simulink model "pingtai_with_control_gaijin1PIDNN3_2"  (R2014a)
settings: Solver=ode23t  StartTime=0.0  StopTime=100.0  MaxStep=1e-2  RelTol=1e-3
values from neighbouring files (symbols this model uses):
  m = 0    [cs_search.m]    (also in pso_search.m = n)
  s = new_nest(j,:)    [empty_nests.m]    (also in get_cuckoos.m = s+stepsize.*randn(size(s)); pso_search.m = newnest(i,:); simplebounds.m = ns_tmp)
undefined symbols (not defined in the file or in its folder): mpidnn, sigbuilder_block, WW, X, Y, Z
libraries: fl_lib x68, sm_lib x65, nesl_utility x65, simulink x18, sm_radial_engine_lib x8, sdl_lib x8, elec_lib x4
(part 4 of 5)

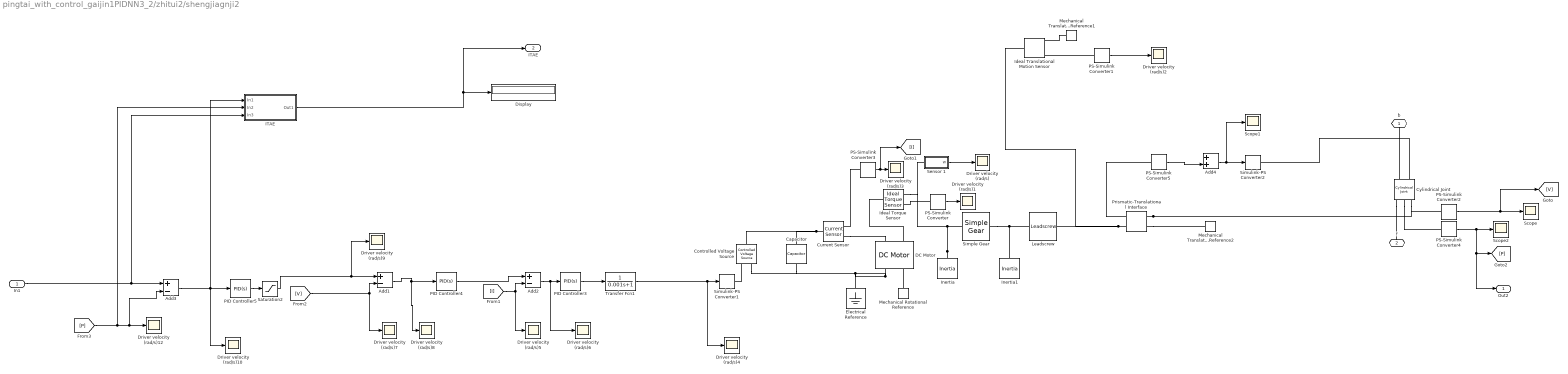
== system pingtai_with_control_gaijin1PIDNN3_2/zhitui2/shengjiagnji2 ==
  In1 : Inport
  "\tITAE" : Subsystem
  Add1 : Sum  Inputs=+-
  Add2 : Sum  Inputs=+-
  Add3 : Sum  Inputs=+-
  Add4 : Sum
  Capacitor : fl_lib/Electrical/Electrical Elements/Capacitor  c=1e-6 F  r=1e-6 Ohm  g=0 1/Ohm  i_specify=off  i_priority=High  i=0 A  v_specify=off  v_priority=High  v=0 V  vc_specify=off  vc_priority=High  vc=0 V
  Controlled Voltage Source : fl_lib/Electrical/Electrical Sources/Controlled Voltage Source
  Current Sensor : fl_lib/Electrical/Electrical Sensors/Current Sensor
  Cylindrical Joint : sm_lib/Joints/Cylindrical Joint  SenseConstraintForce=off  SenseConstraintForceX=off  SenseConstraintForceY=off  SenseConstraintForceZ=off  SenseConstraintTorque=off  SenseConstraintTorqueX=off  SenseConstraintTorqueY=off  SenseConstraintTorqueZ=off  SenseTotalForce=off  SenseTotalForceX=off  SenseTotalForceY=off  SenseTotalForceZ=off  SenseTotalTorque=off  SenseTotalTorqueX=off  SenseTotalTorqueY=off  SenseTotalTorqueZ=off  CompositeWrenchDir=FollowerOnBase  CompositeWrenchFrame=BaseFrame  PzEquilibriumPosition=0  PzEquilibriumPositionUnits=m  PzSpringStiffness=0  PzSpringStiffnessUnits=N/m  PzDampingCoefficient=0  PzDampingCoefficientUnits=N/(m/s)  PzTorqueActuationMode=InputTorque  PzMotionActuationMode=ComputedMotion  PzSensePosition=on  PzSenseVelocity=on  PzSenseAcceleration=off  PzSenseTorqueForce=off  PzPositionTargetValue=init_P  PzPositionTargetValueUnits=m  PzPositionTargetSpecify=on  PzPositionTargetPriority=Low  PzVelocityTargetValue=0  PzVelocityTargetValueUnits=m/s  PzVelocityTargetSpecify=off  PzVelocityTargetPriority=High  RzEquilibriumPosition=0  RzEquilibriumPositionUnits=deg  RzSpringStiffness=0  RzSpringStiffnessUnits=N*m/deg  RzDampingCoefficient=0  RzDampingCoefficientUnits=N*m/(deg/s)  RzTorqueActuationMode=NoTorque  RzMotionActuationMode=ComputedMotion  RzSensePosition=off  RzSenseVelocity=off  RzSenseAcceleration=off  RzSenseTorqueForce=off  RzPositionTargetValue=0  RzPositionTargetValueUnits=deg  RzPositionTargetSpecify=off  RzPositionTargetPriority=High  RzVelocityTargetValue=0  RzVelocityTargetValueUnits=deg/s  RzVelocityTargetSpecify=off  RzVelocityTargetPriority=High  BlockFunction=simmechanics.library.joints.cylindrical_joint
  DC Motor : elec_lib/Actuators & Drivers/Rotational Actuators/DC Motor  parameterization=1  Ra=2 Ohm  La=1.2e-5 H  emf_or_torque=2  Kv=7.2e-5 V/rpm  Ki=6.876e-1 N*m/A  T_stall=2.4e-4 N*m  w_max=1.91e+4 rpm  w_rated=1.5e+4 rpm  P_rated=0.08 W  V_rated=1.5 V  J=0.01 kg*m^2  lam_param=1  lam=0.01 N*m/(rad/s)  i_noload=0 A  V_i_noload=1.5 V  speed0=0 rpm  alpha=0.00393 1/K  Tmeas=25 C  thermal_mass=100 J/K  initial_temperature=25 C
  Display : Display
  Driver velocity (rad/s){,1..10,12} (12 alike) : Scope
      Driver velocity (rad/s) settings: TimeRange=100  YMin=-2  YMax=2  MaxDataPoints=50000
      Driver velocity (rad/s)1 settings: TimeRange=2000  YMin=0  YMax=0.4  SaveName=ScopeData2  MaxDataPoints=50000
      Driver velocity (rad/s)10 settings: TimeRange=50  YMin=-12.5  YMax=15  SaveName=ScopeData12  MaxDataPoints=50000
      Driver velocity (rad/s)12 settings: TimeRange=100  YMin=-20  YMax=120  SaveName=ScopeData19  MaxDataPoints=50000
      Driver velocity (rad/s)2 settings: TimeRange=100  YMin=-2  YMax=2  MaxDataPoints=50000
      Driver velocity (rad/s)3 settings: TimeRange=9.999999999999999e-05  YMin=5.55112e-17  YMax=1.3  SaveName=ScopeData4  MaxDataPoints=50000
      Driver velocity (rad/s)4 settings: TimeRange=20  YMin=395  YMax=460  SaveName=ScopeData7  MaxDataPoints=50000
      Driver velocity (rad/s)5 settings: TimeRange=0.1983737977758173  YMin=65.95890410958904  YMax=71.02739726027397  SaveName=ScopeData5  MaxDataPoints=50000
      Driver velocity (rad/s)6 settings: TimeRange=50  YMin=-12.5  YMax=15  SaveName=ScopeData9  MaxDataPoints=50000
      Driver velocity (rad/s)7 settings: TimeRange=0.7830114694637786  YMin=83.44178082191777  YMax=104.2979452054794  SaveName=ScopeData10  MaxDataPoints=50000
      Driver velocity (rad/s)8 settings: TimeRange=50  YMin=-12.5  YMax=15  SaveName=ScopeData11  MaxDataPoints=50000
      Driver velocity (rad/s)9 settings: TimeRange=20  YMin=76  YMax=84  SaveName=ScopeData30  MaxDataPoints=50000
  Electrical Reference : fl_lib/Electrical/Electrical Elements/Electrical Reference
  Ideal Torque Sensor : fl_lib/Mechanical/Mechanical Sensors/Ideal Torque Sensor
  Ideal Translational Motion Sensor : fl_lib/Mechanical/Mechanical Sensors/Ideal Translational Motion Sensor  offset=0 m
  Inertia : fl_lib/Mechanical/Rotational Elements/Inertia  inertia=0.01 kg*m^2  w_specify=on  w_priority=High  w=0 rad/s  t_specify=off  t_priority=High  t=0 N*m
  Inertia1 : fl_lib/Mechanical/Rotational Elements/Inertia  inertia=0.01 kg*m^2  w_specify=on  w_priority=High  w=0 rad/s  t_specify=off  t_priority=High  t=0 N*m
  Leadscrew : sdl_lib/Gears/Rotational- Translational/Leadscrew  Lead=0.1 m  helix_type=1  friction_model=1  friction_parameterization=1  lambda=15 deg  alpha=14.5 deg  fr_coeff=0.08  eff_sn=0.75  eff_ns=0.45  mu_visc=5 N*m/(rad/s)  v_thr=0.001 m/s
  Mechanical Translational Reference1 : fl_lib/Mechanical/Translational Elements/Mechanical Translational Reference
  Mechanical Translational Reference2 : fl_lib/Mechanical/Translational Elements/Mechanical Translational Reference
  Mechanical Rotational Reference : fl_lib/Mechanical/Rotational Elements/Mechanical Rotational Reference
  PID Controller3 : simulink/Continuous/PID Controller  Controller=PID  TimeDomain=Continuous-time  SampleTime=0.001  IntegratorMethod=Forward Euler  FilterMethod=Forward Euler  Form=Parallel  P=100  I=50000  D=0  N=100  InitialConditionSource=internal  InitialConditionForIntegrator=0  InitialConditionForFilter=0  ExternalReset=none  LimitOutput=off  UpperSaturationLimit=500  LowerSaturationLimit=-500  LinearizeAsGain=on  AntiWindupMode=none  Kb=1  TrackingMode=off  Kt=1  PParamMin=[]  PParamMax=[]  IParamMin=[]  IParamMax=[]  DParamMin=[]  DParamMax=[]  NParamMin=[]  NParamMax=[]  KbParamMin=[]  KbParamMax=[]  KtParamMin=[]  KtParamMax=[]  POutMin=[]  POutMax=[]  IOutMin=[]  IOutMax=[]  DOutMin=[]  DOutMax=[]  NOutMin=[]  NOutMax=[]  KbOutMin=[]  KbOutMax=[]  KtOutMin=[]  KtOutMax=[]  IntegratorOutMin=[]  IntegratorOutMax=[]  FilterOutMin=[]  FilterOutMax=[]  SumOutMin=[]  SumOutMax=[]  SumI1OutMin=[]  SumI1OutMax=[]  SumI2OutMin=[]  SumI2OutMax=[]  SumI3OutMin=[]  SumI3OutMax=[]  SumDOutMin=[]  SumDOutMax=[]  SaturationOutMin=[]  SaturationOutMax=[]  IntegratorContinuousStateAttributes=''  IntegratorStateMustResolveToSignalObject=off  IntegratorRTWStateStorageClass=Auto  FilterContinuousStateAttributes=''  FilterStateMustResolveToSignalObject=off  FilterRTWStateStorageClass=Auto
  PID Controller4 : simulink/Continuous/PID Controller  Controller=PID  TimeDomain=Continuous-time  SampleTime=1  IntegratorMethod=Forward Euler  FilterMethod=Forward Euler  Form=Parallel  P=10  I=18  D=0  N=100  InitialConditionSource=internal  InitialConditionForIntegrator=0  InitialConditionForFilter=0  ExternalReset=none  LimitOutput=off  UpperSaturationLimit=inf  LowerSaturationLimit=-inf  LinearizeAsGain=on  AntiWindupMode=none  Kb=1  TrackingMode=off  Kt=1  PParamMin=[]  PParamMax=[]  IParamMin=[]  IParamMax=[]  DParamMin=[]  DParamMax=[]  NParamMin=[]  NParamMax=[]  KbParamMin=[]  KbParamMax=[]  KtParamMin=[]  KtParamMax=[]  POutMin=[]  POutMax=[]  IOutMin=[]  IOutMax=[]  DOutMin=[]  DOutMax=[]  NOutMin=[]  NOutMax=[]  KbOutMin=[]  KbOutMax=[]  KtOutMin=[]  KtOutMax=[]  IntegratorOutMin=[]  IntegratorOutMax=[]  FilterOutMin=[]  FilterOutMax=[]  SumOutMin=[]  SumOutMax=[]  SumI1OutMin=[]  SumI1OutMax=[]  SumI2OutMin=[]  SumI2OutMax=[]  SumI3OutMin=[]  SumI3OutMax=[]  SumDOutMin=[]  SumDOutMax=[]  SaturationOutMin=[]  SaturationOutMax=[]  IntegratorContinuousStateAttributes=''  IntegratorStateMustResolveToSignalObject=off  IntegratorRTWStateStorageClass=Auto  FilterContinuousStateAttributes=''  FilterStateMustResolveToSignalObject=off  FilterRTWStateStorageClass=Auto
  PID Controller5 : simulink/Continuous/PID Controller  Controller=PID  TimeDomain=Continuous-time  SampleTime=1  IntegratorMethod=Forward Euler  FilterMethod=Forward Euler  Form=Parallel  P=1  I=0  D=0  N=100  InitialConditionSource=internal  InitialConditionForIntegrator=0  InitialConditionForFilter=0  ExternalReset=none  LimitOutput=off  UpperSaturationLimit=inf  LowerSaturationLimit=-inf  LinearizeAsGain=on  AntiWindupMode=none  Kb=1  TrackingMode=off  Kt=1  PParamMin=[]  PParamMax=[]  IParamMin=[]  IParamMax=[]  DParamMin=[]  DParamMax=[]  NParamMin=[]  NParamMax=[]  KbParamMin=[]  KbParamMax=[]  KtParamMin=[]  KtParamMax=[]  POutMin=[]  POutMax=[]  IOutMin=[]  IOutMax=[]  DOutMin=[]  DOutMax=[]  NOutMin=[]  NOutMax=[]  KbOutMin=[]  KbOutMax=[]  KtOutMin=[]  KtOutMax=[]  IntegratorOutMin=[]  IntegratorOutMax=[]  FilterOutMin=[]  FilterOutMax=[]  SumOutMin=[]  SumOutMax=[]  SumI1OutMin=[]  SumI1OutMax=[]  SumI2OutMin=[]  SumI2OutMax=[]  SumI3OutMin=[]  SumI3OutMax=[]  SumDOutMin=[]  SumDOutMax=[]  SaturationOutMin=[]  SaturationOutMax=[]  IntegratorContinuousStateAttributes=''  IntegratorStateMustResolveToSignalObject=off  IntegratorRTWStateStorageClass=Auto  FilterContinuousStateAttributes=''  FilterStateMustResolveToSignalObject=off  FilterRTWStateStorageClass=Auto
  PS-Simulink Converter : nesl_utility/PS-Simulink Converter  PhysicalDomain=network_engine_domain  SubClassName=ps_output  LeftPortType=input  RightPortType=output  PseudoPeriodic=off  Frequencies=[]  Unit=1  AffineConversion=off
  PS-Simulink Converter1 : nesl_utility/PS-Simulink Converter  PhysicalDomain=network_engine_domain  SubClassName=ps_output  LeftPortType=input  RightPortType=output  PseudoPeriodic=off  Frequencies=[]  Unit=m  AffineConversion=off
  PS-Simulink Converter3 : nesl_utility/PS-Simulink Converter  PhysicalDomain=network_engine_domain  SubClassName=ps_output  LeftPortType=input  RightPortType=output  PseudoPeriodic=off  Frequencies=[]  Unit=A  AffineConversion=off
  PS-Simulink Converter2 : nesl_utility/PS-Simulink Converter  PhysicalDomain=network_engine_domain  SubClassName=ps_output  LeftPortType=input  RightPortType=output  PseudoPeriodic=off  Frequencies=[]  Unit=mm/s  AffineConversion=off
  PS-Simulink Converter4 : nesl_utility/PS-Simulink Converter  PhysicalDomain=network_engine_domain  SubClassName=ps_output  LeftPortType=input  RightPortType=output  PseudoPeriodic=off  Frequencies=[]  Unit=mm  AffineConversion=off
  PS-Simulink Converter5 : nesl_utility/PS-Simulink Converter  PhysicalDomain=network_engine_domain  SubClassName=ps_output  LeftPortType=input  RightPortType=output  PseudoPeriodic=off  Frequencies=[]  Unit=N  AffineConversion=off
  Prismatic-Translational Interface : sm_radial_engine_lib/Pneumatic Cylinder Force Model/Prismatic-Translational Interface
  Saturation2 : Saturate  UpperLimit=40  LowerLimit=-40  ZeroCross=off
  Scope : Scope
      settings: TimeRange=20  YMax=25  SaveName=ScopeData3
  Scope1 : Scope
      settings: TimeRange=20  YMin=0.00658085  YMax=0.00727357  SaveName=ScopeData6
  Scope2 : Scope
      settings: TimeRange=20  YMin=0.0998  YMax=0.100225  SaveName=ScopeData8
  Sensor 1 : Subsystem
  Simple Gear : sdl_lib/Gears/Simple Gear  ratio=70  rotation_direction=2  friction_model=1  T_noload=0.1 N*m  T_nom=5 N*m  efficiency_nom=0.8  efficiency=0.8  mu_visc=[ 0 0 ] N*m/(rad/s)  w_thr=0.01 rad/s
  Simulink-PS Converter1 : nesl_utility/Simulink-PS Converter  PhysicalDomain=network_engine_domain  SubClassName=ps_input  LeftPortType=input  RightPortType=output  PseudoPeriodic=off  Frequencies=[]  NoiseDistribution=none  NoiseParameters=[]  Unit=V  AffineConversion=off  InputFiltering=off  SimscapeFilterOrder=2  InputFilterTimeConstant=1  UdotUserProvided=1
  Simulink-PS Converter2 : nesl_utility/Simulink-PS Converter  PhysicalDomain=network_engine_domain  SubClassName=ps_input  LeftPortType=input  RightPortType=output  PseudoPeriodic=off  Frequencies=[]  NoiseDistribution=none  NoiseParameters=[]  Unit=N  AffineConversion=off  InputFiltering=off  SimscapeFilterOrder=2  InputFilterTimeConstant=1  UdotUserProvided=1
  Transfer Fcn1 : TransferFcn  Denominator=[0.001 1]
  b : PMIOPort  Port=1  Side=Right
  f : PMIOPort  Port=2  Side=Right
  Out2 : Outport
  ITAE : Outport  Port=2
  wires:
  Transfer Fcn1/1 -> Simulink-PS Converter1/1, Driver velocity (rad/s)4/1
  Saturation2/1 -> Add1/1, Driver velocity (rad/s)9/1
  PID Controller4/1 -> Add2/1
  In1/1 -> Add3/1, "\tITAE"/3(In3)
  PID Controller5/1 -> Saturation2/1
  [P] -> Add3/2, Driver velocity (rad/s)12/1, "\tITAE"/2(In2)
  Add3/1 -> Driver velocity (rad/s)10/1, "\tITAE"/1(In1), PID Controller5/1
  [V] -> Add1/2, Driver velocity (rad/s)7/1
  Add1/1 -> Driver velocity (rad/s)8/1, PID Controller4/1
  PS-Simulink Converter2/1 -> [V], Scope/1
  PS-Simulink Converter4/1 -> [P], Out2/1, Scope2/1
  PS-Simulink Converter5/1 -> Add4/2
  Add4/1 -> Simulink-PS Converter2/1, Scope1/1
  [I] -> Add2/2, Driver velocity (rad/s)5/1
  "\tITAE"/1(Out1) -> Display/1, ITAE/1
  PID Controller3/1 -> Transfer Fcn1/1
  Add2/1 -> Driver velocity (rad/s)6/1, PID Controller3/1
  PS-Simulink Converter3/1 -> Driver velocity (rad/s)3/1, [I]
  PS-Simulink Converter1/1 -> Driver velocity (rad/s)2/1
  PS-Simulink Converter/1 -> Driver velocity (rad/s)1/1
  Sensor 1/1(w) -> Driver velocity (rad/s)/1
  connections:
  Cylindrical Joint/RConn1 -- f/RConn1
  Cylindrical Joint/LConn1 -- b/RConn1
  Cylindrical Joint/RConn2 -- PS-Simulink Converter4/LConn1
  Cylindrical Joint/LConn2 -- Simulink-PS Converter2/RConn1
  PS-Simulink Converter5/LConn1 -- Prismatic-Translational Interface/RConn1
  Current Sensor/LConn1 -- Controlled Voltage Source/LConn1 -- Capacitor/LConn1
  Prismatic-Translational Interface/RConn2 -- Leadscrew/RConn1 -- Ideal Translational Motion Sensor/LConn1
  PS-Simulink Converter3/LConn1 -- Current Sensor/RConn1
  Prismatic-Translational Interface/LConn2 -- Mechanical Translational Reference2/LConn1
  Mechanical Translational Reference1/LConn1 -- Ideal Translational Motion Sensor/RConn1
  PS-Simulink Converter1/LConn1 -- Ideal Translational Motion Sensor/RConn3
  Ideal Torque Sensor/RConn2 -- PS-Simulink Converter/LConn1
  DC Motor/LConn2 -- Ideal Torque Sensor/LConn1
  Simulink-PS Converter1/RConn1 -- Controlled Voltage Source/RConn1
  Current Sensor/RConn2 -- DC Motor/LConn1
  Inertia1/LConn1 -- Simple Gear/RConn1 -- Leadscrew/LConn1
  Inertia/LConn1 -- Simple Gear/LConn1 -- Ideal Torque Sensor/RConn1 -- Sensor 1/LConn1
  Mechanical Rotational Reference/LConn1 -- DC Motor/RConn2
  DC Motor/RConn1 -- Electrical Reference/LConn1 -- Capacitor/RConn1 -- Controlled Voltage Source/RConn2
  Prismatic-Translational Interface/LConn1 -- Cylindrical Joint/RConn3 -- PS-Simulink Converter2/LConn1

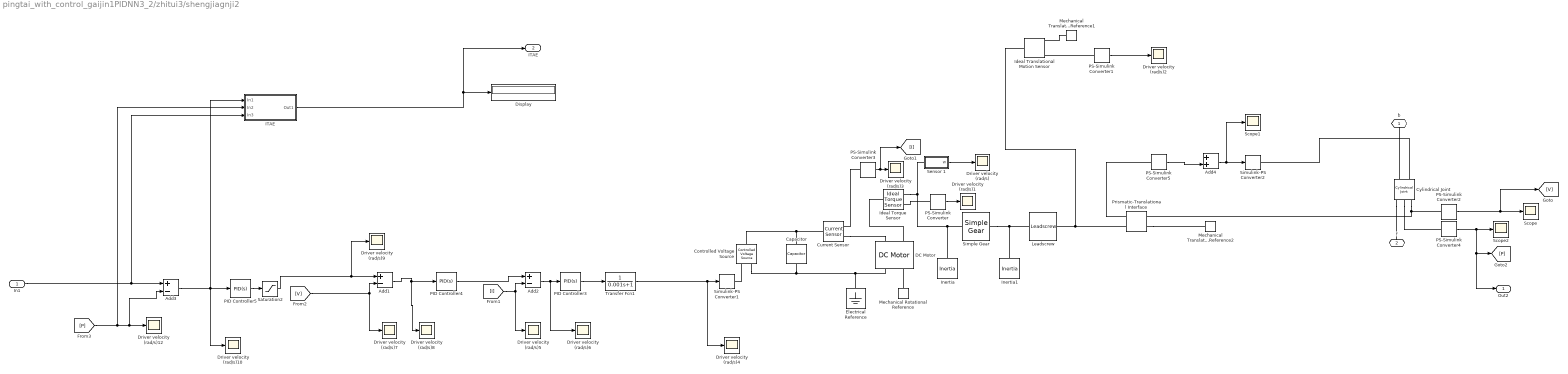
== system pingtai_with_control_gaijin1PIDNN3_2/zhitui3/shengjiagnji2 ==
  In1 : Inport
  "\tITAE" : Subsystem
  Add1 : Sum  Inputs=+-
  Add2 : Sum  Inputs=+-
  Add3 : Sum  Inputs=+-
  Add4 : Sum
  Capacitor : fl_lib/Electrical/Electrical Elements/Capacitor  c=1e-6 F  r=1e-6 Ohm  g=0 1/Ohm  i_specify=off  i_priority=High  i=0 A  v_specify=off  v_priority=High  v=0 V  vc_specify=off  vc_priority=High  vc=0 V
  Controlled Voltage Source : fl_lib/Electrical/Electrical Sources/Controlled Voltage Source
  Current Sensor : fl_lib/Electrical/Electrical Sensors/Current Sensor
  Cylindrical Joint : sm_lib/Joints/Cylindrical Joint  SenseConstraintForce=off  SenseConstraintForceX=off  SenseConstraintForceY=off  SenseConstraintForceZ=off  SenseConstraintTorque=off  SenseConstraintTorqueX=off  SenseConstraintTorqueY=off  SenseConstraintTorqueZ=off  SenseTotalForce=off  SenseTotalForceX=off  SenseTotalForceY=off  SenseTotalForceZ=off  SenseTotalTorque=off  SenseTotalTorqueX=off  SenseTotalTorqueY=off  SenseTotalTorqueZ=off  CompositeWrenchDir=FollowerOnBase  CompositeWrenchFrame=BaseFrame  PzEquilibriumPosition=0  PzEquilibriumPositionUnits=m  PzSpringStiffness=0  PzSpringStiffnessUnits=N/m  PzDampingCoefficient=0  PzDampingCoefficientUnits=N/(m/s)  PzTorqueActuationMode=InputTorque  PzMotionActuationMode=ComputedMotion  PzSensePosition=on  PzSenseVelocity=on  PzSenseAcceleration=off  PzSenseTorqueForce=off  PzPositionTargetValue=init_P  PzPositionTargetValueUnits=m  PzPositionTargetSpecify=on  PzPositionTargetPriority=Low  PzVelocityTargetValue=0  PzVelocityTargetValueUnits=m/s  PzVelocityTargetSpecify=off  PzVelocityTargetPriority=High  RzEquilibriumPosition=0  RzEquilibriumPositionUnits=deg  RzSpringStiffness=0  RzSpringStiffnessUnits=N*m/deg  RzDampingCoefficient=0  RzDampingCoefficientUnits=N*m/(deg/s)  RzTorqueActuationMode=NoTorque  RzMotionActuationMode=ComputedMotion  RzSensePosition=off  RzSenseVelocity=off  RzSenseAcceleration=off  RzSenseTorqueForce=off  RzPositionTargetValue=0  RzPositionTargetValueUnits=deg  RzPositionTargetSpecify=off  RzPositionTargetPriority=High  RzVelocityTargetValue=0  RzVelocityTargetValueUnits=deg/s  RzVelocityTargetSpecify=off  RzVelocityTargetPriority=High  BlockFunction=simmechanics.library.joints.cylindrical_joint
  DC Motor : elec_lib/Actuators & Drivers/Rotational Actuators/DC Motor  parameterization=1  Ra=2 Ohm  La=1.2e-5 H  emf_or_torque=2  Kv=7.2e-5 V/rpm  Ki=6.876e-1 N*m/A  T_stall=2.4e-4 N*m  w_max=1.91e+4 rpm  w_rated=1.5e+4 rpm  P_rated=0.08 W  V_rated=1.5 V  J=0.01 kg*m^2  lam_param=1  lam=0.01 N*m/(rad/s)  i_noload=0 A  V_i_noload=1.5 V  speed0=0 rpm  alpha=0.00393 1/K  Tmeas=25 C  thermal_mass=100 J/K  initial_temperature=25 C
  Display : Display
  Driver velocity (rad/s){,1..10,12} (12 alike) : Scope
      Driver velocity (rad/s) settings: TimeRange=100  YMin=-2  YMax=2  MaxDataPoints=50000
      Driver velocity (rad/s)1 settings: TimeRange=2000  YMin=0  YMax=0.4  SaveName=ScopeData2  MaxDataPoints=50000
      Driver velocity (rad/s)10 settings: TimeRange=50  YMin=-12.5  YMax=15  SaveName=ScopeData12  MaxDataPoints=50000
      Driver velocity (rad/s)12 settings: TimeRange=100  YMin=-20  YMax=120  SaveName=ScopeData19  MaxDataPoints=50000
      Driver velocity (rad/s)2 settings: TimeRange=100  YMin=-2  YMax=2  MaxDataPoints=50000
      Driver velocity (rad/s)3 settings: TimeRange=9.999999999999999e-05  YMin=5.55112e-17  YMax=1.3  SaveName=ScopeData4  MaxDataPoints=50000
      Driver velocity (rad/s)4 settings: TimeRange=20  YMin=395  YMax=460  SaveName=ScopeData7  MaxDataPoints=50000
      Driver velocity (rad/s)5 settings: TimeRange=0.1983737977758173  YMin=65.95890410958904  YMax=71.02739726027397  SaveName=ScopeData5  MaxDataPoints=50000
      Driver velocity (rad/s)6 settings: TimeRange=50  YMin=-12.5  YMax=15  SaveName=ScopeData9  MaxDataPoints=50000
      Driver velocity (rad/s)7 settings: TimeRange=0.7830114694637786  YMin=83.44178082191777  YMax=104.2979452054794  SaveName=ScopeData10  MaxDataPoints=50000
      Driver velocity (rad/s)8 settings: TimeRange=50  YMin=-12.5  YMax=15  SaveName=ScopeData11  MaxDataPoints=50000
      Driver velocity (rad/s)9 settings: TimeRange=20  YMin=76  YMax=84  SaveName=ScopeData30  MaxDataPoints=50000
  Electrical Reference : fl_lib/Electrical/Electrical Elements/Electrical Reference
  Ideal Torque Sensor : fl_lib/Mechanical/Mechanical Sensors/Ideal Torque Sensor
  Ideal Translational Motion Sensor : fl_lib/Mechanical/Mechanical Sensors/Ideal Translational Motion Sensor  offset=0 m
  Inertia : fl_lib/Mechanical/Rotational Elements/Inertia  inertia=0.01 kg*m^2  w_specify=on  w_priority=High  w=0 rad/s  t_specify=off  t_priority=High  t=0 N*m
  Inertia1 : fl_lib/Mechanical/Rotational Elements/Inertia  inertia=0.01 kg*m^2  w_specify=on  w_priority=High  w=0 rad/s  t_specify=off  t_priority=High  t=0 N*m
  Leadscrew : sdl_lib/Gears/Rotational- Translational/Leadscrew  Lead=0.1 m  helix_type=1  friction_model=1  friction_parameterization=1  lambda=15 deg  alpha=14.5 deg  fr_coeff=0.08  eff_sn=0.75  eff_ns=0.45  mu_visc=5 N*m/(rad/s)  v_thr=0.001 m/s
  Mechanical Translational Reference1 : fl_lib/Mechanical/Translational Elements/Mechanical Translational Reference
  Mechanical Translational Reference2 : fl_lib/Mechanical/Translational Elements/Mechanical Translational Reference
  Mechanical Rotational Reference : fl_lib/Mechanical/Rotational Elements/Mechanical Rotational Reference
  PID Controller3 : simulink/Continuous/PID Controller  Controller=PID  TimeDomain=Continuous-time  SampleTime=0.001  IntegratorMethod=Forward Euler  FilterMethod=Forward Euler  Form=Parallel  P=100  I=50000  D=0  N=100  InitialConditionSource=internal  InitialConditionForIntegrator=0  InitialConditionForFilter=0  ExternalReset=none  LimitOutput=off  UpperSaturationLimit=500  LowerSaturationLimit=-500  LinearizeAsGain=on  AntiWindupMode=none  Kb=1  TrackingMode=off  Kt=1  PParamMin=[]  PParamMax=[]  IParamMin=[]  IParamMax=[]  DParamMin=[]  DParamMax=[]  NParamMin=[]  NParamMax=[]  KbParamMin=[]  KbParamMax=[]  KtParamMin=[]  KtParamMax=[]  POutMin=[]  POutMax=[]  IOutMin=[]  IOutMax=[]  DOutMin=[]  DOutMax=[]  NOutMin=[]  NOutMax=[]  KbOutMin=[]  KbOutMax=[]  KtOutMin=[]  KtOutMax=[]  IntegratorOutMin=[]  IntegratorOutMax=[]  FilterOutMin=[]  FilterOutMax=[]  SumOutMin=[]  SumOutMax=[]  SumI1OutMin=[]  SumI1OutMax=[]  SumI2OutMin=[]  SumI2OutMax=[]  SumI3OutMin=[]  SumI3OutMax=[]  SumDOutMin=[]  SumDOutMax=[]  SaturationOutMin=[]  SaturationOutMax=[]  IntegratorContinuousStateAttributes=''  IntegratorStateMustResolveToSignalObject=off  IntegratorRTWStateStorageClass=Auto  FilterContinuousStateAttributes=''  FilterStateMustResolveToSignalObject=off  FilterRTWStateStorageClass=Auto
  PID Controller4 : simulink/Continuous/PID Controller  Controller=PID  TimeDomain=Continuous-time  SampleTime=1  IntegratorMethod=Forward Euler  FilterMethod=Forward Euler  Form=Parallel  P=10  I=18  D=0  N=100  InitialConditionSource=internal  InitialConditionForIntegrator=0  InitialConditionForFilter=0  ExternalReset=none  LimitOutput=off  UpperSaturationLimit=inf  LowerSaturationLimit=-inf  LinearizeAsGain=on  AntiWindupMode=none  Kb=1  TrackingMode=off  Kt=1  PParamMin=[]  PParamMax=[]  IParamMin=[]  IParamMax=[]  DParamMin=[]  DParamMax=[]  NParamMin=[]  NParamMax=[]  KbParamMin=[]  KbParamMax=[]  KtParamMin=[]  KtParamMax=[]  POutMin=[]  POutMax=[]  IOutMin=[]  IOutMax=[]  DOutMin=[]  DOutMax=[]  NOutMin=[]  NOutMax=[]  KbOutMin=[]  KbOutMax=[]  KtOutMin=[]  KtOutMax=[]  IntegratorOutMin=[]  IntegratorOutMax=[]  FilterOutMin=[]  FilterOutMax=[]  SumOutMin=[]  SumOutMax=[]  SumI1OutMin=[]  SumI1OutMax=[]  SumI2OutMin=[]  SumI2OutMax=[]  SumI3OutMin=[]  SumI3OutMax=[]  SumDOutMin=[]  SumDOutMax=[]  SaturationOutMin=[]  SaturationOutMax=[]  IntegratorContinuousStateAttributes=''  IntegratorStateMustResolveToSignalObject=off  IntegratorRTWStateStorageClass=Auto  FilterContinuousStateAttributes=''  FilterStateMustResolveToSignalObject=off  FilterRTWStateStorageClass=Auto
  PID Controller5 : simulink/Continuous/PID Controller  Controller=PID  TimeDomain=Continuous-time  SampleTime=1  IntegratorMethod=Forward Euler  FilterMethod=Forward Euler  Form=Parallel  P=1  I=0  D=0  N=100  InitialConditionSource=internal  InitialConditionForIntegrator=0  InitialConditionForFilter=0  ExternalReset=none  LimitOutput=off  UpperSaturationLimit=inf  LowerSaturationLimit=-inf  LinearizeAsGain=on  AntiWindupMode=none  Kb=1  TrackingMode=off  Kt=1  PParamMin=[]  PParamMax=[]  IParamMin=[]  IParamMax=[]  DParamMin=[]  DParamMax=[]  NParamMin=[]  NParamMax=[]  KbParamMin=[]  KbParamMax=[]  KtParamMin=[]  KtParamMax=[]  POutMin=[]  POutMax=[]  IOutMin=[]  IOutMax=[]  DOutMin=[]  DOutMax=[]  NOutMin=[]  NOutMax=[]  KbOutMin=[]  KbOutMax=[]  KtOutMin=[]  KtOutMax=[]  IntegratorOutMin=[]  IntegratorOutMax=[]  FilterOutMin=[]  FilterOutMax=[]  SumOutMin=[]  SumOutMax=[]  SumI1OutMin=[]  SumI1OutMax=[]  SumI2OutMin=[]  SumI2OutMax=[]  SumI3OutMin=[]  SumI3OutMax=[]  SumDOutMin=[]  SumDOutMax=[]  SaturationOutMin=[]  SaturationOutMax=[]  IntegratorContinuousStateAttributes=''  IntegratorStateMustResolveToSignalObject=off  IntegratorRTWStateStorageClass=Auto  FilterContinuousStateAttributes=''  FilterStateMustResolveToSignalObject=off  FilterRTWStateStorageClass=Auto
  PS-Simulink Converter : nesl_utility/PS-Simulink Converter  PhysicalDomain=network_engine_domain  SubClassName=ps_output  LeftPortType=input  RightPortType=output  PseudoPeriodic=off  Frequencies=[]  Unit=1  AffineConversion=off
  PS-Simulink Converter1 : nesl_utility/PS-Simulink Converter  PhysicalDomain=network_engine_domain  SubClassName=ps_output  LeftPortType=input  RightPortType=output  PseudoPeriodic=off  Frequencies=[]  Unit=m  AffineConversion=off
  PS-Simulink Converter3 : nesl_utility/PS-Simulink Converter  PhysicalDomain=network_engine_domain  SubClassName=ps_output  LeftPortType=input  RightPortType=output  PseudoPeriodic=off  Frequencies=[]  Unit=A  AffineConversion=off
  PS-Simulink Converter2 : nesl_utility/PS-Simulink Converter  PhysicalDomain=network_engine_domain  SubClassName=ps_output  LeftPortType=input  RightPortType=output  PseudoPeriodic=off  Frequencies=[]  Unit=mm/s  AffineConversion=off
  PS-Simulink Converter4 : nesl_utility/PS-Simulink Converter  PhysicalDomain=network_engine_domain  SubClassName=ps_output  LeftPortType=input  RightPortType=output  PseudoPeriodic=off  Frequencies=[]  Unit=mm  AffineConversion=off
  PS-Simulink Converter5 : nesl_utility/PS-Simulink Converter  PhysicalDomain=network_engine_domain  SubClassName=ps_output  LeftPortType=input  RightPortType=output  PseudoPeriodic=off  Frequencies=[]  Unit=N  AffineConversion=off
  Prismatic-Translational Interface : sm_radial_engine_lib/Pneumatic Cylinder Force Model/Prismatic-Translational Interface
  Saturation2 : Saturate  UpperLimit=40  LowerLimit=-40  ZeroCross=off
  Scope : Scope
      settings: TimeRange=20  YMax=25  SaveName=ScopeData3
  Scope1 : Scope
      settings: TimeRange=20  YMin=0.00658085  YMax=0.00727357  SaveName=ScopeData6
  Scope2 : Scope
      settings: TimeRange=20  YMin=0.0998  YMax=0.100225  SaveName=ScopeData8
  Sensor 1 : Subsystem
  Simple Gear : sdl_lib/Gears/Simple Gear  ratio=70  rotation_direction=2  friction_model=1  T_noload=0.1 N*m  T_nom=5 N*m  efficiency_nom=0.8  efficiency=0.8  mu_visc=[ 0 0 ] N*m/(rad/s)  w_thr=0.01 rad/s
  Simulink-PS Converter1 : nesl_utility/Simulink-PS Converter  PhysicalDomain=network_engine_domain  SubClassName=ps_input  LeftPortType=input  RightPortType=output  PseudoPeriodic=off  Frequencies=[]  NoiseDistribution=none  NoiseParameters=[]  Unit=V  AffineConversion=off  InputFiltering=off  SimscapeFilterOrder=2  InputFilterTimeConstant=1  UdotUserProvided=1
  Simulink-PS Converter2 : nesl_utility/Simulink-PS Converter  PhysicalDomain=network_engine_domain  SubClassName=ps_input  LeftPortType=input  RightPortType=output  PseudoPeriodic=off  Frequencies=[]  NoiseDistribution=none  NoiseParameters=[]  Unit=N  AffineConversion=off  InputFiltering=off  SimscapeFilterOrder=2  InputFilterTimeConstant=1  UdotUserProvided=1
  Transfer Fcn1 : TransferFcn  Denominator=[0.001 1]
  b : PMIOPort  Port=1  Side=Right
  f : PMIOPort  Port=2  Side=Right
  Out2 : Outport
  ITAE : Outport  Port=2
  wires:
  Sensor 1/1(w) -> Driver velocity (rad/s)/1
  PS-Simulink Converter/1 -> Driver velocity (rad/s)1/1
  PS-Simulink Converter1/1 -> Driver velocity (rad/s)2/1
  PS-Simulink Converter3/1 -> [I], Driver velocity (rad/s)3/1
  Add2/1 -> PID Controller3/1, Driver velocity (rad/s)6/1
  PID Controller3/1 -> Transfer Fcn1/1
  "\tITAE"/1(Out1) -> ITAE/1, Display/1
  [I] -> Driver velocity (rad/s)5/1, Add2/2
  Add4/1 -> Scope1/1, Simulink-PS Converter2/1
  PS-Simulink Converter5/1 -> Add4/2
  PS-Simulink Converter4/1 -> Scope2/1, Out2/1, [P]
  PS-Simulink Converter2/1 -> Scope/1, [V]
  Add1/1 -> PID Controller4/1, Driver velocity (rad/s)8/1
  [V] -> Driver velocity (rad/s)7/1, Add1/2
  Add3/1 -> PID Controller5/1, "\tITAE"/1(In1), Driver velocity (rad/s)10/1
  [P] -> "\tITAE"/2(In2), Driver velocity (rad/s)12/1, Add3/2
  PID Controller5/1 -> Saturation2/1
  In1/1 -> "\tITAE"/3(In3), Add3/1
  PID Controller4/1 -> Add2/1
  Saturation2/1 -> Driver velocity (rad/s)9/1, Add1/1
  Transfer Fcn1/1 -> Driver velocity (rad/s)4/1, Simulink-PS Converter1/1
  connections:
  PS-Simulink Converter2/LConn1 -- Cylindrical Joint/RConn3 -- Prismatic-Translational Interface/LConn1
  Controlled Voltage Source/RConn2 -- Capacitor/RConn1 -- Electrical Reference/LConn1 -- DC Motor/RConn1
  Mechanical Rotational Reference/LConn1 -- DC Motor/RConn2
  Sensor 1/LConn1 -- Ideal Torque Sensor/RConn1 -- Simple Gear/LConn1 -- Inertia/LConn1
  Leadscrew/LConn1 -- Simple Gear/RConn1 -- Inertia1/LConn1
  Current Sensor/RConn2 -- DC Motor/LConn1
  Simulink-PS Converter1/RConn1 -- Controlled Voltage Source/RConn1
  DC Motor/LConn2 -- Ideal Torque Sensor/LConn1
  Ideal Torque Sensor/RConn2 -- PS-Simulink Converter/LConn1
  PS-Simulink Converter1/LConn1 -- Ideal Translational Motion Sensor/RConn3
  Mechanical Translational Reference1/LConn1 -- Ideal Translational Motion Sensor/RConn1
  Prismatic-Translational Interface/LConn2 -- Mechanical Translational Reference2/LConn1
  PS-Simulink Converter3/LConn1 -- Current Sensor/RConn1
  Ideal Translational Motion Sensor/LConn1 -- Leadscrew/RConn1 -- Prismatic-Translational Interface/RConn2
  Capacitor/LConn1 -- Controlled Voltage Source/LConn1 -- Current Sensor/LConn1
  PS-Simulink Converter5/LConn1 -- Prismatic-Translational Interface/RConn1
  Cylindrical Joint/LConn2 -- Simulink-PS Converter2/RConn1
  Cylindrical Joint/RConn2 -- PS-Simulink Converter4/LConn1
  Cylindrical Joint/LConn1 -- b/RConn1
  Cylindrical Joint/RConn1 -- f/RConn1

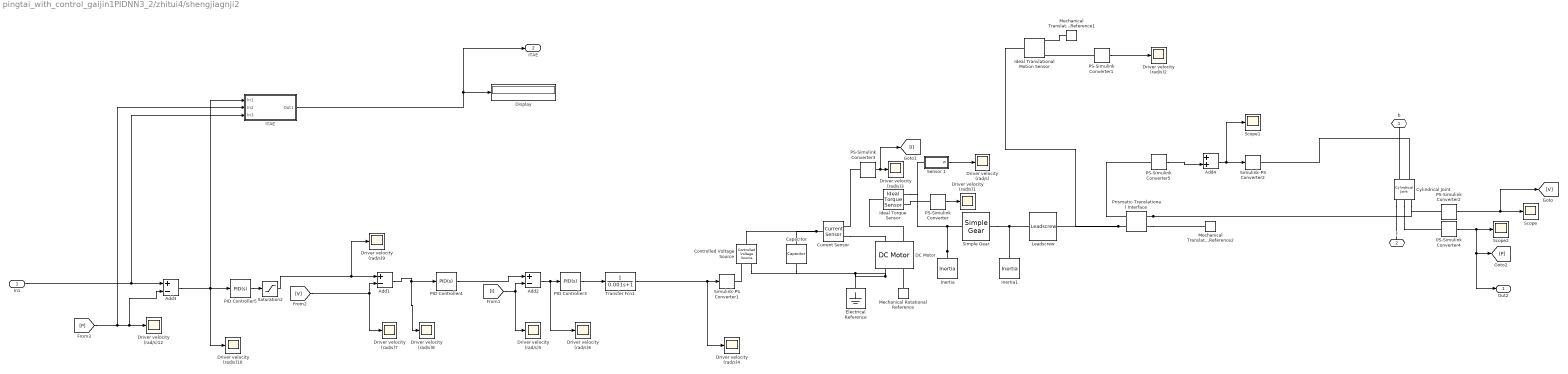
== system pingtai_with_control_gaijin1PIDNN3_2/zhitui4/shengjiagnji2 ==
  In1 : Inport
  "\tITAE" : Subsystem
  Add1 : Sum  Inputs=+-
  Add2 : Sum  Inputs=+-
  Add3 : Sum  Inputs=+-
  Add4 : Sum
  Capacitor : fl_lib/Electrical/Electrical Elements/Capacitor  c=1e-6 F  r=1e-6 Ohm  g=0 1/Ohm  i_specify=off  i_priority=High  i=0 A  v_specify=off  v_priority=High  v=0 V  vc_specify=off  vc_priority=High  vc=0 V
  Controlled Voltage Source : fl_lib/Electrical/Electrical Sources/Controlled Voltage Source
  Current Sensor : fl_lib/Electrical/Electrical Sensors/Current Sensor
  Cylindrical Joint : sm_lib/Joints/Cylindrical Joint  SenseConstraintForce=off  SenseConstraintForceX=off  SenseConstraintForceY=off  SenseConstraintForceZ=off  SenseConstraintTorque=off  SenseConstraintTorqueX=off  SenseConstraintTorqueY=off  SenseConstraintTorqueZ=off  SenseTotalForce=off  SenseTotalForceX=off  SenseTotalForceY=off  SenseTotalForceZ=off  SenseTotalTorque=off  SenseTotalTorqueX=off  SenseTotalTorqueY=off  SenseTotalTorqueZ=off  CompositeWrenchDir=FollowerOnBase  CompositeWrenchFrame=BaseFrame  PzEquilibriumPosition=0  PzEquilibriumPositionUnits=m  PzSpringStiffness=0  PzSpringStiffnessUnits=N/m  PzDampingCoefficient=0  PzDampingCoefficientUnits=N/(m/s)  PzTorqueActuationMode=InputTorque  PzMotionActuationMode=ComputedMotion  PzSensePosition=on  PzSenseVelocity=on  PzSenseAcceleration=off  PzSenseTorqueForce=off  PzPositionTargetValue=init_P  PzPositionTargetValueUnits=m  PzPositionTargetSpecify=on  PzPositionTargetPriority=Low  PzVelocityTargetValue=0  PzVelocityTargetValueUnits=m/s  PzVelocityTargetSpecify=off  PzVelocityTargetPriority=High  RzEquilibriumPosition=0  RzEquilibriumPositionUnits=deg  RzSpringStiffness=0  RzSpringStiffnessUnits=N*m/deg  RzDampingCoefficient=0  RzDampingCoefficientUnits=N*m/(deg/s)  RzTorqueActuationMode=NoTorque  RzMotionActuationMode=ComputedMotion  RzSensePosition=off  RzSenseVelocity=off  RzSenseAcceleration=off  RzSenseTorqueForce=off  RzPositionTargetValue=0  RzPositionTargetValueUnits=deg  RzPositionTargetSpecify=off  RzPositionTargetPriority=High  RzVelocityTargetValue=0  RzVelocityTargetValueUnits=deg/s  RzVelocityTargetSpecify=off  RzVelocityTargetPriority=High  BlockFunction=simmechanics.library.joints.cylindrical_joint
  DC Motor : elec_lib/Actuators & Drivers/Rotational Actuators/DC Motor  parameterization=1  Ra=2 Ohm  La=1.2e-5 H  emf_or_torque=2  Kv=7.2e-5 V/rpm  Ki=6.876e-1 N*m/A  T_stall=2.4e-4 N*m  w_max=1.91e+4 rpm  w_rated=1.5e+4 rpm  P_rated=0.08 W  V_rated=1.5 V  J=0.01 kg*m^2  lam_param=1  lam=0.01 N*m/(rad/s)  i_noload=0 A  V_i_noload=1.5 V  speed0=0 rpm  alpha=0.00393 1/K  Tmeas=25 C  thermal_mass=100 J/K  initial_temperature=25 C
  Display : Display
  Driver velocity (rad/s){,1..10,12} (12 alike) : Scope
      Driver velocity (rad/s) settings: TimeRange=100  YMin=-2  YMax=2  MaxDataPoints=50000
      Driver velocity (rad/s)1 settings: TimeRange=2000  YMin=0  YMax=0.4  SaveName=ScopeData2  MaxDataPoints=50000
      Driver velocity (rad/s)10 settings: TimeRange=50  YMin=-12.5  YMax=15  SaveName=ScopeData12  MaxDataPoints=50000
      Driver velocity (rad/s)12 settings: TimeRange=100  YMin=-20  YMax=120  SaveName=ScopeData19  MaxDataPoints=50000
      Driver velocity (rad/s)2 settings: TimeRange=100  YMin=-2  YMax=2  MaxDataPoints=50000
      Driver velocity (rad/s)3 settings: TimeRange=9.999999999999999e-05  YMin=5.55112e-17  YMax=1.3  SaveName=ScopeData4  MaxDataPoints=50000
      Driver velocity (rad/s)4 settings: TimeRange=20  YMin=395  YMax=460  SaveName=ScopeData7  MaxDataPoints=50000
      Driver velocity (rad/s)5 settings: TimeRange=0.1983737977758173  YMin=65.95890410958904  YMax=71.02739726027397  SaveName=ScopeData5  MaxDataPoints=50000
      Driver velocity (rad/s)6 settings: TimeRange=50  YMin=-12.5  YMax=15  SaveName=ScopeData9  MaxDataPoints=50000
      Driver velocity (rad/s)7 settings: TimeRange=0.7830114694637786  YMin=83.44178082191777  YMax=104.2979452054794  SaveName=ScopeData10  MaxDataPoints=50000
      Driver velocity (rad/s)8 settings: TimeRange=50  YMin=-12.5  YMax=15  SaveName=ScopeData11  MaxDataPoints=50000
      Driver velocity (rad/s)9 settings: TimeRange=20  YMin=76  YMax=84  SaveName=ScopeData30  MaxDataPoints=50000
  Electrical Reference : fl_lib/Electrical/Electrical Elements/Electrical Reference
  Ideal Torque Sensor : fl_lib/Mechanical/Mechanical Sensors/Ideal Torque Sensor
  Ideal Translational Motion Sensor : fl_lib/Mechanical/Mechanical Sensors/Ideal Translational Motion Sensor  offset=0 m
  Inertia : fl_lib/Mechanical/Rotational Elements/Inertia  inertia=0.01 kg*m^2  w_specify=on  w_priority=High  w=0 rad/s  t_specify=off  t_priority=High  t=0 N*m
  Inertia1 : fl_lib/Mechanical/Rotational Elements/Inertia  inertia=0.01 kg*m^2  w_specify=on  w_priority=High  w=0 rad/s  t_specify=off  t_priority=High  t=0 N*m
  Leadscrew : sdl_lib/Gears/Rotational- Translational/Leadscrew  Lead=0.1 m  helix_type=1  friction_model=1  friction_parameterization=1  lambda=15 deg  alpha=14.5 deg  fr_coeff=0.08  eff_sn=0.75  eff_ns=0.45  mu_visc=5 N*m/(rad/s)  v_thr=0.001 m/s
  Mechanical Translational Reference1 : fl_lib/Mechanical/Translational Elements/Mechanical Translational Reference
  Mechanical Translational Reference2 : fl_lib/Mechanical/Translational Elements/Mechanical Translational Reference
  Mechanical Rotational Reference : fl_lib/Mechanical/Rotational Elements/Mechanical Rotational Reference
  PID Controller3 : simulink/Continuous/PID Controller  Controller=PID  TimeDomain=Continuous-time  SampleTime=0.001  IntegratorMethod=Forward Euler  FilterMethod=Forward Euler  Form=Parallel  P=100  I=50000  D=0  N=100  InitialConditionSource=internal  InitialConditionForIntegrator=0  InitialConditionForFilter=0  ExternalReset=none  LimitOutput=off  UpperSaturationLimit=500  LowerSaturationLimit=-500  LinearizeAsGain=on  AntiWindupMode=none  Kb=1  TrackingMode=off  Kt=1  PParamMin=[]  PParamMax=[]  IParamMin=[]  IParamMax=[]  DParamMin=[]  DParamMax=[]  NParamMin=[]  NParamMax=[]  KbParamMin=[]  KbParamMax=[]  KtParamMin=[]  KtParamMax=[]  POutMin=[]  POutMax=[]  IOutMin=[]  IOutMax=[]  DOutMin=[]  DOutMax=[]  NOutMin=[]  NOutMax=[]  KbOutMin=[]  KbOutMax=[]  KtOutMin=[]  KtOutMax=[]  IntegratorOutMin=[]  IntegratorOutMax=[]  FilterOutMin=[]  FilterOutMax=[]  SumOutMin=[]  SumOutMax=[]  SumI1OutMin=[]  SumI1OutMax=[]  SumI2OutMin=[]  SumI2OutMax=[]  SumI3OutMin=[]  SumI3OutMax=[]  SumDOutMin=[]  SumDOutMax=[]  SaturationOutMin=[]  SaturationOutMax=[]  IntegratorContinuousStateAttributes=''  IntegratorStateMustResolveToSignalObject=off  IntegratorRTWStateStorageClass=Auto  FilterContinuousStateAttributes=''  FilterStateMustResolveToSignalObject=off  FilterRTWStateStorageClass=Auto
  PID Controller4 : simulink/Continuous/PID Controller  Controller=PID  TimeDomain=Continuous-time  SampleTime=1  IntegratorMethod=Forward Euler  FilterMethod=Forward Euler  Form=Parallel  P=10  I=18  D=0  N=100  InitialConditionSource=internal  InitialConditionForIntegrator=0  InitialConditionForFilter=0  ExternalReset=none  LimitOutput=off  UpperSaturationLimit=inf  LowerSaturationLimit=-inf  LinearizeAsGain=on  AntiWindupMode=none  Kb=1  TrackingMode=off  Kt=1  PParamMin=[]  PParamMax=[]  IParamMin=[]  IParamMax=[]  DParamMin=[]  DParamMax=[]  NParamMin=[]  NParamMax=[]  KbParamMin=[]  KbParamMax=[]  KtParamMin=[]  KtParamMax=[]  POutMin=[]  POutMax=[]  IOutMin=[]  IOutMax=[]  DOutMin=[]  DOutMax=[]  NOutMin=[]  NOutMax=[]  KbOutMin=[]  KbOutMax=[]  KtOutMin=[]  KtOutMax=[]  IntegratorOutMin=[]  IntegratorOutMax=[]  FilterOutMin=[]  FilterOutMax=[]  SumOutMin=[]  SumOutMax=[]  SumI1OutMin=[]  SumI1OutMax=[]  SumI2OutMin=[]  SumI2OutMax=[]  SumI3OutMin=[]  SumI3OutMax=[]  SumDOutMin=[]  SumDOutMax=[]  SaturationOutMin=[]  SaturationOutMax=[]  IntegratorContinuousStateAttributes=''  IntegratorStateMustResolveToSignalObject=off  IntegratorRTWStateStorageClass=Auto  FilterContinuousStateAttributes=''  FilterStateMustResolveToSignalObject=off  FilterRTWStateStorageClass=Auto
  PID Controller5 : simulink/Continuous/PID Controller  Controller=PID  TimeDomain=Continuous-time  SampleTime=1  IntegratorMethod=Forward Euler  FilterMethod=Forward Euler  Form=Parallel  P=1  I=0  D=0  N=100  InitialConditionSource=internal  InitialConditionForIntegrator=0  InitialConditionForFilter=0  ExternalReset=none  LimitOutput=off  UpperSaturationLimit=inf  LowerSaturationLimit=-inf  LinearizeAsGain=on  AntiWindupMode=none  Kb=1  TrackingMode=off  Kt=1  PParamMin=[]  PParamMax=[]  IParamMin=[]  IParamMax=[]  DParamMin=[]  DParamMax=[]  NParamMin=[]  NParamMax=[]  KbParamMin=[]  KbParamMax=[]  KtParamMin=[]  KtParamMax=[]  POutMin=[]  POutMax=[]  IOutMin=[]  IOutMax=[]  DOutMin=[]  DOutMax=[]  NOutMin=[]  NOutMax=[]  KbOutMin=[]  KbOutMax=[]  KtOutMin=[]  KtOutMax=[]  IntegratorOutMin=[]  IntegratorOutMax=[]  FilterOutMin=[]  FilterOutMax=[]  SumOutMin=[]  SumOutMax=[]  SumI1OutMin=[]  SumI1OutMax=[]  SumI2OutMin=[]  SumI2OutMax=[]  SumI3OutMin=[]  SumI3OutMax=[]  SumDOutMin=[]  SumDOutMax=[]  SaturationOutMin=[]  SaturationOutMax=[]  IntegratorContinuousStateAttributes=''  IntegratorStateMustResolveToSignalObject=off  IntegratorRTWStateStorageClass=Auto  FilterContinuousStateAttributes=''  FilterStateMustResolveToSignalObject=off  FilterRTWStateStorageClass=Auto
  PS-Simulink Converter : nesl_utility/PS-Simulink Converter  PhysicalDomain=network_engine_domain  SubClassName=ps_output  LeftPortType=input  RightPortType=output  PseudoPeriodic=off  Frequencies=[]  Unit=1  AffineConversion=off
  PS-Simulink Converter1 : nesl_utility/PS-Simulink Converter  PhysicalDomain=network_engine_domain  SubClassName=ps_output  LeftPortType=input  RightPortType=output  PseudoPeriodic=off  Frequencies=[]  Unit=m  AffineConversion=off
  PS-Simulink Converter3 : nesl_utility/PS-Simulink Converter  PhysicalDomain=network_engine_domain  SubClassName=ps_output  LeftPortType=input  RightPortType=output  PseudoPeriodic=off  Frequencies=[]  Unit=A  AffineConversion=off
  PS-Simulink Converter2 : nesl_utility/PS-Simulink Converter  PhysicalDomain=network_engine_domain  SubClassName=ps_output  LeftPortType=input  RightPortType=output  PseudoPeriodic=off  Frequencies=[]  Unit=mm/s  AffineConversion=off
  PS-Simulink Converter4 : nesl_utility/PS-Simulink Converter  PhysicalDomain=network_engine_domain  SubClassName=ps_output  LeftPortType=input  RightPortType=output  PseudoPeriodic=off  Frequencies=[]  Unit=mm  AffineConversion=off
  PS-Simulink Converter5 : nesl_utility/PS-Simulink Converter  PhysicalDomain=network_engine_domain  SubClassName=ps_output  LeftPortType=input  RightPortType=output  PseudoPeriodic=off  Frequencies=[]  Unit=N  AffineConversion=off
  Prismatic-Translational Interface : sm_radial_engine_lib/Pneumatic Cylinder Force Model/Prismatic-Translational Interface
  Saturation2 : Saturate  UpperLimit=40  LowerLimit=-40  ZeroCross=off
  Scope : Scope
      settings: TimeRange=20  YMax=25  SaveName=ScopeData3
  Scope1 : Scope
      settings: TimeRange=20  YMin=0.00658085  YMax=0.00727357  SaveName=ScopeData6
  Scope2 : Scope
      settings: TimeRange=20  YMin=0.0998  YMax=0.100225  SaveName=ScopeData8
  Sensor 1 : Subsystem
  Simple Gear : sdl_lib/Gears/Simple Gear  ratio=70  rotation_direction=2  friction_model=1  T_noload=0.1 N*m  T_nom=5 N*m  efficiency_nom=0.8  efficiency=0.8  mu_visc=[ 0 0 ] N*m/(rad/s)  w_thr=0.01 rad/s
  Simulink-PS Converter1 : nesl_utility/Simulink-PS Converter  PhysicalDomain=network_engine_domain  SubClassName=ps_input  LeftPortType=input  RightPortType=output  PseudoPeriodic=off  Frequencies=[]  NoiseDistribution=none  NoiseParameters=[]  Unit=V  AffineConversion=off  InputFiltering=off  SimscapeFilterOrder=2  InputFilterTimeConstant=1  UdotUserProvided=1
  Simulink-PS Converter2 : nesl_utility/Simulink-PS Converter  PhysicalDomain=network_engine_domain  SubClassName=ps_input  LeftPortType=input  RightPortType=output  PseudoPeriodic=off  Frequencies=[]  NoiseDistribution=none  NoiseParameters=[]  Unit=N  AffineConversion=off  InputFiltering=off  SimscapeFilterOrder=2  InputFilterTimeConstant=1  UdotUserProvided=1
  Transfer Fcn1 : TransferFcn  Denominator=[0.001 1]
  b : PMIOPort  Port=1  Side=Right
  f : PMIOPort  Port=2  Side=Right
  Out2 : Outport
  ITAE : Outport  Port=2
  wires:
  Transfer Fcn1/1 -> Simulink-PS Converter1/1, Driver velocity (rad/s)4/1
  Saturation2/1 -> Add1/1, Driver velocity (rad/s)9/1
  PID Controller4/1 -> Add2/1
  In1/1 -> Add3/1, "\tITAE"/3(In3)
  PID Controller5/1 -> Saturation2/1
  [P] -> Add3/2, Driver velocity (rad/s)12/1, "\tITAE"/2(In2)
  Add3/1 -> Driver velocity (rad/s)10/1, "\tITAE"/1(In1), PID Controller5/1
  [V] -> Add1/2, Driver velocity (rad/s)7/1
  Add1/1 -> Driver velocity (rad/s)8/1, PID Controller4/1
  PS-Simulink Converter2/1 -> [V], Scope/1
  PS-Simulink Converter4/1 -> [P], Out2/1, Scope2/1
  PS-Simulink Converter5/1 -> Add4/2
  Add4/1 -> Simulink-PS Converter2/1, Scope1/1
  [I] -> Add2/2, Driver velocity (rad/s)5/1
  "\tITAE"/1(Out1) -> Display/1, ITAE/1
  PID Controller3/1 -> Transfer Fcn1/1
  Add2/1 -> Driver velocity (rad/s)6/1, PID Controller3/1
  PS-Simulink Converter3/1 -> Driver velocity (rad/s)3/1, [I]
  PS-Simulink Converter1/1 -> Driver velocity (rad/s)2/1
  PS-Simulink Converter/1 -> Driver velocity (rad/s)1/1
  Sensor 1/1(w) -> Driver velocity (rad/s)/1
  connections:
  Cylindrical Joint/RConn1 -- f/RConn1
  Cylindrical Joint/LConn1 -- b/RConn1
  Cylindrical Joint/RConn2 -- PS-Simulink Converter4/LConn1
  Cylindrical Joint/LConn2 -- Simulink-PS Converter2/RConn1
  PS-Simulink Converter5/LConn1 -- Prismatic-Translational Interface/RConn1
  Current Sensor/LConn1 -- Controlled Voltage Source/LConn1 -- Capacitor/LConn1
  Prismatic-Translational Interface/RConn2 -- Leadscrew/RConn1 -- Ideal Translational Motion Sensor/LConn1
  PS-Simulink Converter3/LConn1 -- Current Sensor/RConn1
  Prismatic-Translational Interface/LConn2 -- Mechanical Translational Reference2/LConn1
  Mechanical Translational Reference1/LConn1 -- Ideal Translational Motion Sensor/RConn1
  PS-Simulink Converter1/LConn1 -- Ideal Translational Motion Sensor/RConn3
  Ideal Torque Sensor/RConn2 -- PS-Simulink Converter/LConn1
  DC Motor/LConn2 -- Ideal Torque Sensor/LConn1
  Simulink-PS Converter1/RConn1 -- Controlled Voltage Source/RConn1
  Current Sensor/RConn2 -- DC Motor/LConn1
  Inertia1/LConn1 -- Simple Gear/RConn1 -- Leadscrew/LConn1
  Inertia/LConn1 -- Simple Gear/LConn1 -- Ideal Torque Sensor/RConn1 -- Sensor 1/LConn1
  Mechanical Rotational Reference/LConn1 -- DC Motor/RConn2
  DC Motor/RConn1 -- Electrical Reference/LConn1 -- Capacitor/RConn1 -- Controlled Voltage Source/RConn2
  Prismatic-Translational Interface/LConn1 -- Cylindrical Joint/RConn3 -- PS-Simulink Converter2/LConn1

== system pingtai_with_control_gaijin1PIDNN3_2/zhitui1/shengjiagnji2/	ITAE ==
  In1 : Inport
  In2 : Inport  Port=2
  In3 : Inport  Port=3
  Abs : Abs  ZeroCross=off  SaturateOnIntegerOverflow=on
  Add : Sum  Inputs=+-
  Add1 : Sum
  Display : Display
  Display1 : Display
  Gain : Gain  Gain=50
  Gain1 : Gain  Gain=80
  Integrator1 : Integrator
  MinMax Running Resettable : simulink/Math Operations/MinMax Running Resettable  Function=max  vinit=0.0
  Product1 : Product  SaturateOnIntegerOverflow=on  OutDataTypeStr=Inherit: Same as first input
  time : Clock
  Out1 : Outport
  wires:
  time/1 -> Product1/1
  Integrator1/1 -> Gain/1, Display/1
  Product1/1 -> Integrator1/1
  Abs/1 -> Product1/2
  In1/1 -> Abs/1
  Add/1 -> MinMax Running Resettable/1
  MinMax Running Resettable/1 -> Gain1/1, Display1/1
  In2/1 -> Add/1
  In3/1 -> Add/2
  Gain/1 -> Add1/1
  Gain1/1 -> Add1/2
  Add1/1 -> Out1/1

== system pingtai_with_control_gaijin1PIDNN3_2/zhitui1/shengjiagnji2/Sensor 1 ==
  Ideal Rotational Motion Sensor : fl_lib/Mechanical/Mechanical Sensors/Ideal Rotational Motion Sensor  offset=0 rad
  MRR3 : fl_lib/Mechanical/Rotational Elements/Mechanical Rotational Reference
  PS-Simulink Converter : nesl_utility/PS-Simulink Converter  PhysicalDomain=network_engine_domain  SubClassName=ps_output  LeftPortType=input  RightPortType=output  PseudoPeriodic=off  Frequencies=[]  Unit=1  AffineConversion=off
  R : PMIOPort  Port=1  Side=Left
  w : Outport
  wires:
  PS-Simulink Converter/1 -> w/1
  connections:
  MRR3/LConn1 -- Ideal Rotational Motion Sensor/RConn1
  Ideal Rotational Motion Sensor/RConn2 -- PS-Simulink Converter/LConn1
  R/RConn1 -- Ideal Rotational Motion Sensor/LConn1

== system pingtai_with_control_gaijin1PIDNN3_2/zhitui2/shengjiagnji2/	ITAE ==
  In1 : Inport
  In2 : Inport  Port=2
  In3 : Inport  Port=3
  Abs : Abs  ZeroCross=off  SaturateOnIntegerOverflow=on
  Add : Sum  Inputs=+-
  Add1 : Sum
  Display : Display
  Display1 : Display
  Gain : Gain  Gain=50
  Gain1 : Gain  Gain=80
  Integrator1 : Integrator
  MinMax Running Resettable : simulink/Math Operations/MinMax Running Resettable  Function=max  vinit=0.0
  Product1 : Product  SaturateOnIntegerOverflow=on  OutDataTypeStr=Inherit: Same as first input
  time : Clock
  Out1 : Outport
  wires:
  Add1/1 -> Out1/1
  Gain1/1 -> Add1/2
  Gain/1 -> Add1/1
  In3/1 -> Add/2
  In2/1 -> Add/1
  MinMax Running Resettable/1 -> Display1/1, Gain1/1
  Add/1 -> MinMax Running Resettable/1
  In1/1 -> Abs/1
  Abs/1 -> Product1/2
  Product1/1 -> Integrator1/1
  Integrator1/1 -> Display/1, Gain/1
  time/1 -> Product1/1

== system pingtai_with_control_gaijin1PIDNN3_2/zhitui2/shengjiagnji2/Sensor 1 ==
  Ideal Rotational Motion Sensor : fl_lib/Mechanical/Mechanical Sensors/Ideal Rotational Motion Sensor  offset=0 rad
  MRR3 : fl_lib/Mechanical/Rotational Elements/Mechanical Rotational Reference
  PS-Simulink Converter : nesl_utility/PS-Simulink Converter  PhysicalDomain=network_engine_domain  SubClassName=ps_output  LeftPortType=input  RightPortType=output  PseudoPeriodic=off  Frequencies=[]  Unit=1  AffineConversion=off
  R : PMIOPort  Port=1  Side=Left
  w : Outport
  wires:
  PS-Simulink Converter/1 -> w/1
  connections:
  R/RConn1 -- Ideal Rotational Motion Sensor/LConn1
  Ideal Rotational Motion Sensor/RConn2 -- PS-Simulink Converter/LConn1
  MRR3/LConn1 -- Ideal Rotational Motion Sensor/RConn1

== system pingtai_with_control_gaijin1PIDNN3_2/zhitui3/shengjiagnji2/	ITAE ==
  In1 : Inport
  In2 : Inport  Port=2
  In3 : Inport  Port=3
  Abs : Abs  ZeroCross=off  SaturateOnIntegerOverflow=on
  Add : Sum  Inputs=+-
  Add1 : Sum
  Display : Display
  Display1 : Display
  Gain : Gain  Gain=50
  Gain1 : Gain  Gain=80
  Integrator1 : Integrator
  MinMax Running Resettable : simulink/Math Operations/MinMax Running Resettable  Function=max  vinit=0.0
  Product1 : Product  SaturateOnIntegerOverflow=on  OutDataTypeStr=Inherit: Same as first input
  time : Clock
  Out1 : Outport
  wires:
  time/1 -> Product1/1
  Integrator1/1 -> Gain/1, Display/1
  Product1/1 -> Integrator1/1
  Abs/1 -> Product1/2
  In1/1 -> Abs/1
  Add/1 -> MinMax Running Resettable/1
  MinMax Running Resettable/1 -> Gain1/1, Display1/1
  In2/1 -> Add/1
  In3/1 -> Add/2
  Gain/1 -> Add1/1
  Gain1/1 -> Add1/2
  Add1/1 -> Out1/1
